simulink model "case7"  (R2024b)
settings: Solver=FixedStepAuto  StartTime=0  StopTime=1  FixedStep=1e-7  RelTol=1e-3
values from neighbouring files (symbols this model uses):
  SG_D_1_D = 0.01056    [IEEE9_case_parameters.m]    (also in case1_parameters.m; case2_parameters.m; case3_parameters.m; case4_parameters.m)
  SG_D_1_EnableSaturation = 0    [IEEE9_case_parameters.m]    (also in case1_parameters.m; case2_parameters.m; case3_parameters.m; case4_parameters.m)
  SG_D_1_f0 = 60    [IEEE9_case_parameters.m]    (also in case1_parameters.m; case2_parameters.m; case3_parameters.m; case4_parameters.m)
  SG_D_1_H = 7.5    [IEEE9_case_parameters.m]    (also in case1_parameters.m; case2_parameters.m; case3_parameters.m; case4_parameters.m)
  SG_D_1_K_A = 20    [IEEE9_case_parameters.m]    (also in case1_parameters.m; case2_parameters.m; case3_parameters.m; case4_parameters.m)
  SG_D_1_K_E = 1.000000e+1    (= 10)    [IEEE9_case_parameters.m]    (also in case1_parameters.m; case2_parameters.m; case3_parameters.m; case4_parameters.m)
  SG_D_1_K_F = 2.363    [IEEE9_case_parameters.m]    (also in case1_parameters.m; case2_parameters.m; case3_parameters.m; case4_parameters.m)
  SG_D_1_K_s = 0.5    [IEEE9_case_parameters.m]    (also in case1_parameters.m = 5; case2_parameters.m = 5; case3_parameters.m = 5; case4_parameters.m = 5)
  SG_D_1_R_a = 0.001088    [IEEE9_case_parameters.m]    (also in case1_parameters.m; case2_parameters.m; case3_parameters.m; case4_parameters.m)
  SG_D_1_S_A = 1    [IEEE9_case_parameters.m]    (also in case1_parameters.m; case2_parameters.m; case3_parameters.m; case4_parameters.m)
  SG_D_1_S_B = 0.103    [IEEE9_case_parameters.m]    (also in case1_parameters.m; case2_parameters.m; case3_parameters.m; case4_parameters.m)
  SG_D_1_S_N = 10.659857    [IEEE9_case_parameters.m]    (also in case1_parameters.m; case2_parameters.m; case3_parameters.m; case4_parameters.m)
  SG_D_1_SpeedPara = 200    [IEEE9_case_parameters.m]    (also in case1_parameters.m; case2_parameters.m; case3_parameters.m; case4_parameters.m)
  SG_D_1_T_0 = 0.720173    [IEEE9_case_parameters.m]    (also in case1_parameters.m = 0.755522; case2_parameters.m = 0.808931; case3_parameters.m = 0.869402; case4_parameters.m = 0.729316)
  SG_D_1_T_1 = 0.3    [IEEE9_case_parameters.m]    (also in case1_parameters.m; case2_parameters.m; case3_parameters.m; case4_parameters.m)
  SG_D_1_T_2 = 0.05    [IEEE9_case_parameters.m]    (also in case1_parameters.m; case2_parameters.m; case3_parameters.m; case4_parameters.m)
  SG_D_1_T_3 = 0.02    [IEEE9_case_parameters.m]    (also in case1_parameters.m; case2_parameters.m; case3_parameters.m; case4_parameters.m)
  SG_D_1_T_4 = 0.005    [IEEE9_case_parameters.m]    (also in case1_parameters.m; case2_parameters.m; case3_parameters.m; case4_parameters.m)
  SG_D_1_T_A = 0.02    [IEEE9_case_parameters.m]    (also in case1_parameters.m; case2_parameters.m; case3_parameters.m; case4_parameters.m)
  SG_D_1_T_dd = 8.000000e+0    (= 8)    [IEEE9_case_parameters.m]    (also in case1_parameters.m; case2_parameters.m; case3_parameters.m; case4_parameters.m)
  SG_D_1_T_ddd = 0.04    [IEEE9_case_parameters.m]    (also in case1_parameters.m; case2_parameters.m; case3_parameters.m; case4_parameters.m)
  SG_D_1_T_E = 0.314    [IEEE9_case_parameters.m]    (also in case1_parameters.m; case2_parameters.m; case3_parameters.m; case4_parameters.m)
  SG_D_1_T_F = 0.35    [IEEE9_case_parameters.m]    (also in case1_parameters.m; case2_parameters.m; case3_parameters.m; case4_parameters.m)
  SG_D_1_T_qd = 0.8    [IEEE9_case_parameters.m]    (also in case1_parameters.m; case2_parameters.m; case3_parameters.m; case4_parameters.m)
  SG_D_1_T_qdd = 0.02    [IEEE9_case_parameters.m]    (also in case1_parameters.m; case2_parameters.m; case3_parameters.m; case4_parameters.m)
  SG_D_1_T_speed = 0.1    [IEEE9_case_parameters.m]    (also in case1_parameters.m = 200; case2_parameters.m = 200; case3_parameters.m = 200; case4_parameters.m = 200)
  SG_D_1_T_w = 0.5    [IEEE9_case_parameters.m]    (also in case1_parameters.m; case2_parameters.m; case3_parameters.m; case4_parameters.m)
  SG_D_1_V_ref = 1.990276    [IEEE9_case_parameters.m]    (also in case1_parameters.m = 2.042296; case2_parameters.m = 2.051388; case3_parameters.m = 2.089584; case4_parameters.m = 2.01845)
  SG_D_1_w_ref = 376.991118    [IEEE9_case_parameters.m]    (also in case1_parameters.m; case2_parameters.m; case3_parameters.m; case4_parameters.m)
  SG_D_1_wb = 6.000000e+1    (= 60)    [IEEE9_case_parameters.m]    (also in case1_parameters.m; case2_parameters.m; case3_parameters.m; case4_parameters.m)
  SG_D_1_x_d = 1.9    [IEEE9_case_parameters.m]    (also in case1_parameters.m; case2_parameters.m; case3_parameters.m; case4_parameters.m)
  SG_D_1_x_dd = 0.302    [IEEE9_case_parameters.m]    (also in case1_parameters.m; case2_parameters.m; case3_parameters.m; case4_parameters.m)
  SG_D_1_x_ddd = 0.204    [IEEE9_case_parameters.m]    (also in case1_parameters.m; case2_parameters.m; case3_parameters.m; case4_parameters.m)
  SG_D_1_x_l = 0.05    [IEEE9_case_parameters.m]    (also in case1_parameters.m; case2_parameters.m; case3_parameters.m; case4_parameters.m)
  SG_D_1_x_q = 1.3    [IEEE9_case_parameters.m]    (also in case1_parameters.m; case2_parameters.m; case3_parameters.m; case4_parameters.m)
  SG_D_1_x_qd = 0.5    [IEEE9_case_parameters.m]    (also in case1_parameters.m; case2_parameters.m; case3_parameters.m; case4_parameters.m)
  SG_D_1_x_qdd = 0.3    [IEEE9_case_parameters.m]    (also in case1_parameters.m; case2_parameters.m; case3_parameters.m; case4_parameters.m)
  SG_D_2_D = 0.02    [IEEE9_case_parameters.m]    (also in case1_parameters.m; case2_parameters.m; case3_parameters.m; case4_parameters.m)
  SG_D_2_EnableSaturation = 0    [IEEE9_case_parameters.m]    (also in case1_parameters.m; case2_parameters.m; case3_parameters.m; case4_parameters.m)
  SG_D_2_f0 = 60    [IEEE9_case_parameters.m]    (also in case1_parameters.m; case2_parameters.m; case3_parameters.m; case4_parameters.m)
  SG_D_2_H = 8.000000e+0    (= 8)    [IEEE9_case_parameters.m]    (also in case1_parameters.m; case2_parameters.m; case3_parameters.m; case4_parameters.m)
  SG_D_2_K_A = 20    [IEEE9_case_parameters.m]    (also in case1_parameters.m; case2_parameters.m; case3_parameters.m; case4_parameters.m)
  SG_D_2_K_E = 1.000000e+1    (= 10)    [IEEE9_case_parameters.m]    (also in case1_parameters.m; case2_parameters.m; case3_parameters.m; case4_parameters.m)
  SG_D_2_K_F = 2.363    [IEEE9_case_parameters.m]    (also in case1_parameters.m; case2_parameters.m; case3_parameters.m; case4_parameters.m)
  SG_D_2_K_s = 0.5    [IEEE9_case_parameters.m]    (also in case1_parameters.m = 4; case2_parameters.m = 4; case3_parameters.m = 4; case4_parameters.m = 4)
  SG_D_2_R_a = 0.001088    [IEEE9_case_parameters.m]    (also in case1_parameters.m; case2_parameters.m; case3_parameters.m; case4_parameters.m)
  SG_D_2_S_A = 1    [IEEE9_case_parameters.m]    (also in case1_parameters.m; case2_parameters.m; case3_parameters.m; case4_parameters.m)
  SG_D_2_S_B = 0.103    [IEEE9_case_parameters.m]    (also in case1_parameters.m; case2_parameters.m; case3_parameters.m; case4_parameters.m)
  SG_D_2_S_N = 10.659857    [IEEE9_case_parameters.m]    (also in case1_parameters.m; case2_parameters.m; case3_parameters.m; case4_parameters.m)
  SG_D_2_SpeedPara = 200    [IEEE9_case_parameters.m]    (also in case1_parameters.m; case2_parameters.m; case3_parameters.m; case4_parameters.m)
  SG_D_2_T_0 = 1.632913    [IEEE9_case_parameters.m]    (also in case1_parameters.m = 1.632925; case2_parameters.m = 1.632915; case3_parameters.m = 1.632914; case4_parameters.m = 1.632927)
  SG_D_2_T_1 = 0.2    [IEEE9_case_parameters.m]    (also in case1_parameters.m; case2_parameters.m; case3_parameters.m; case4_parameters.m)
  SG_D_2_T_2 = 0.05    [IEEE9_case_parameters.m]    (also in case1_parameters.m; case2_parameters.m; case3_parameters.m; case4_parameters.m)
  SG_D_2_T_3 = 0.02    [IEEE9_case_parameters.m]    (also in case1_parameters.m; case2_parameters.m; case3_parameters.m; case4_parameters.m)
  SG_D_2_T_4 = 0.005    [IEEE9_case_parameters.m]    (also in case1_parameters.m; case2_parameters.m; case3_parameters.m; case4_parameters.m)
  SG_D_2_T_A = 0.02    [IEEE9_case_parameters.m]    (also in case1_parameters.m; case2_parameters.m; case3_parameters.m; case4_parameters.m)
  SG_D_2_T_dd = 7.9    [IEEE9_case_parameters.m]    (also in case1_parameters.m; case2_parameters.m; case3_parameters.m; case4_parameters.m)
  SG_D_2_T_ddd = 0.04    [IEEE9_case_parameters.m]    (also in case1_parameters.m; case2_parameters.m; case3_parameters.m; case4_parameters.m)
  SG_D_2_T_E = 0.314    [IEEE9_case_parameters.m]    (also in case1_parameters.m; case2_parameters.m; case3_parameters.m; case4_parameters.m)
  SG_D_2_T_F = 0.35    [IEEE9_case_parameters.m]    (also in case1_parameters.m; case2_parameters.m; case3_parameters.m; case4_parameters.m)
  SG_D_2_T_qd = 0.8    [IEEE9_case_parameters.m]    (also in case1_parameters.m; case2_parameters.m; case3_parameters.m; case4_parameters.m)
  SG_D_2_T_qdd = 0.015    [IEEE9_case_parameters.m]    (also in case1_parameters.m; case2_parameters.m; case3_parameters.m; case4_parameters.m)
  SG_D_2_T_speed = 0.1    [IEEE9_case_parameters.m]    (also in case1_parameters.m = 150; case2_parameters.m = 150; case3_parameters.m = 150; case4_parameters.m = 150)
  SG_D_2_T_w = 0.35    [IEEE9_case_parameters.m]    (also in case1_parameters.m; case2_parameters.m; case3_parameters.m; case4_parameters.m)
  SG_D_2_V_ref = 2.58547    [IEEE9_case_parameters.m]    (also in case1_parameters.m = 2.597896; case2_parameters.m = 2.587136; case3_parameters.m = 2.586042; case4_parameters.m = 2.599679)
  SG_D_2_w_ref = 376.991118    [IEEE9_case_parameters.m]    (also in case1_parameters.m; case2_parameters.m; case3_parameters.m; case4_parameters.m)
  SG_D_2_wb = 6.000000e+1    (= 60)    [IEEE9_case_parameters.m]    (also in case1_parameters.m; case2_parameters.m; case3_parameters.m; case4_parameters.m)
  SG_D_2_x_d = 1.8    [IEEE9_case_parameters.m]    (also in case1_parameters.m; case2_parameters.m; case3_parameters.m; case4_parameters.m)
  SG_D_2_x_dd = 0.302    [IEEE9_case_parameters.m]    (also in case1_parameters.m; case2_parameters.m; case3_parameters.m; case4_parameters.m)
  SG_D_2_x_ddd = 0.204    [IEEE9_case_parameters.m]    (also in case1_parameters.m; case2_parameters.m; case3_parameters.m; case4_parameters.m)
  SG_D_2_x_l = 0.05    [IEEE9_case_parameters.m]    (also in case1_parameters.m; case2_parameters.m; case3_parameters.m; case4_parameters.m)
  SG_D_2_x_q = 1.25    [IEEE9_case_parameters.m]    (also in case1_parameters.m; case2_parameters.m; case3_parameters.m; case4_parameters.m)
  SG_D_2_x_qd = 0.5    [IEEE9_case_parameters.m]    (also in case1_parameters.m; case2_parameters.m; case3_parameters.m; case4_parameters.m)
  SG_D_2_x_qdd = 0.3    [IEEE9_case_parameters.m]    (also in case1_parameters.m; case2_parameters.m; case3_parameters.m; case4_parameters.m)
  SG_D_3_D = 0.02    [IEEE9_case_parameters.m]    (also in case1_parameters.m; case2_parameters.m; case3_parameters.m; case4_parameters.m)
  SG_D_3_EnableSaturation = 0    [IEEE9_case_parameters.m]    (also in case1_parameters.m; case2_parameters.m; case3_parameters.m; case4_parameters.m)
  SG_D_3_f0 = 60    [IEEE9_case_parameters.m]    (also in case1_parameters.m; case2_parameters.m; case3_parameters.m; case4_parameters.m)
  SG_D_3_H = 7.7    [IEEE9_case_parameters.m]    (also in case1_parameters.m; case2_parameters.m; case3_parameters.m; case4_parameters.m)
  SG_D_3_K_A = 20    [IEEE9_case_parameters.m]    (also in case1_parameters.m; case2_parameters.m; case3_parameters.m; case4_parameters.m)
  SG_D_3_K_E = 1.000000e+1    (= 10)    [IEEE9_case_parameters.m]    (also in case1_parameters.m; case2_parameters.m; case3_parameters.m; case4_parameters.m)
  SG_D_3_K_F = 2.363    [IEEE9_case_parameters.m]    (also in case1_parameters.m; case2_parameters.m; case3_parameters.m; case4_parameters.m)
  SG_D_3_K_s = 0.2    [IEEE9_case_parameters.m]    (also in case1_parameters.m = 2; case2_parameters.m = 2; case3_parameters.m = 2; case4_parameters.m = 2)
  SG_D_3_R_a = 0.001088    [IEEE9_case_parameters.m]    (also in case1_parameters.m; case2_parameters.m; case3_parameters.m; case4_parameters.m)
  SG_D_3_S_A = 1    [IEEE9_case_parameters.m]    (also in case1_parameters.m; case2_parameters.m; case3_parameters.m; case4_parameters.m)
  SG_D_3_S_B = 0.103    [IEEE9_case_parameters.m]    (also in case1_parameters.m; case2_parameters.m; case3_parameters.m; case4_parameters.m)
  SG_D_3_S_N = 10.659857    [IEEE9_case_parameters.m]    (also in case1_parameters.m; case2_parameters.m; case3_parameters.m; case4_parameters.m)
  SG_D_3_SpeedPara = 200    [IEEE9_case_parameters.m]    (also in case1_parameters.m; case2_parameters.m; case3_parameters.m; case4_parameters.m)
  SG_D_3_T_0 = 0.850788    [IEEE9_case_parameters.m]    (also in case1_parameters.m = 0.850786; case2_parameters.m = 0.850787; case3_parameters.m; case4_parameters.m = 0.850786)
  SG_D_3_T_1 = 0.2    [IEEE9_case_parameters.m]    (also in case1_parameters.m; case2_parameters.m; case3_parameters.m; case4_parameters.m)
  SG_D_3_T_2 = 0.05    [IEEE9_case_parameters.m]    (also in case1_parameters.m; case2_parameters.m; case3_parameters.m; case4_parameters.m)
  SG_D_3_T_3 = 0.02    [IEEE9_case_parameters.m]    (also in case1_parameters.m; case2_parameters.m; case3_parameters.m; case4_parameters.m)
  SG_D_3_T_4 = 0.005    [IEEE9_case_parameters.m]    (also in case1_parameters.m; case2_parameters.m; case3_parameters.m; case4_parameters.m)
  SG_D_3_T_A = 0.02    [IEEE9_case_parameters.m]    (also in case1_parameters.m; case2_parameters.m; case3_parameters.m; case4_parameters.m)
  SG_D_3_T_dd = 8.1    [IEEE9_case_parameters.m]    (also in case1_parameters.m; case2_parameters.m; case3_parameters.m; case4_parameters.m)
  SG_D_3_T_ddd = 0.04    [IEEE9_case_parameters.m]    (also in case1_parameters.m; case2_parameters.m; case3_parameters.m; case4_parameters.m)
  SG_D_3_T_E = 0.314    [IEEE9_case_parameters.m]    (also in case1_parameters.m; case2_parameters.m; case3_parameters.m; case4_parameters.m)
  SG_D_3_T_F = 0.35    [IEEE9_case_parameters.m]    (also in case1_parameters.m; case2_parameters.m; case3_parameters.m; case4_parameters.m)
  SG_D_3_T_qd = 0.8    [IEEE9_case_parameters.m]    (also in case1_parameters.m; case2_parameters.m; case3_parameters.m; case4_parameters.m)
  SG_D_3_T_qdd = 0.015    [IEEE9_case_parameters.m]    (also in case1_parameters.m; case2_parameters.m; case3_parameters.m; case4_parameters.m)
  SG_D_3_T_speed = 0.1    [IEEE9_case_parameters.m]    (also in case1_parameters.m = 180; case2_parameters.m = 180; case3_parameters.m = 180; case4_parameters.m = 180)
  SG_D_3_T_w = 0.4    [IEEE9_case_parameters.m]    (also in case1_parameters.m; case2_parameters.m; case3_parameters.m; case4_parameters.m)
  SG_D_3_V_ref = 1.892727    [IEEE9_case_parameters.m]    (also in case1_parameters.m = 1.906439; case2_parameters.m = 1.895535; case3_parameters.m = 1.892105; case4_parameters.m = 1.906598)
  SG_D_3_w_ref = 376.991118    [IEEE9_case_parameters.m]    (also in case1_parameters.m; case2_parameters.m; case3_parameters.m; case4_parameters.m)
  SG_D_3_wb = 6.000000e+1    (= 60)    [IEEE9_case_parameters.m]    (also in case1_parameters.m; case2_parameters.m; case3_parameters.m; case4_parameters.m)
  SG_D_3_x_d = 1.85    [IEEE9_case_parameters.m]    (also in case1_parameters.m; case2_parameters.m; case3_parameters.m; case4_parameters.m)
  SG_D_3_x_dd = 0.302    [IEEE9_case_parameters.m]    (also in case1_parameters.m; case2_parameters.m; case3_parameters.m; case4_parameters.m)
  SG_D_3_x_ddd = 0.204    [IEEE9_case_parameters.m]    (also in case1_parameters.m; case2_parameters.m; case3_parameters.m; case4_parameters.m)
  SG_D_3_x_l = 0.05    [IEEE9_case_parameters.m]    (also in case1_parameters.m; case2_parameters.m; case3_parameters.m; case4_parameters.m)
  SG_D_3_x_q = 1.2    [IEEE9_case_parameters.m]    (also in case1_parameters.m; case2_parameters.m; case3_parameters.m; case4_parameters.m)
  SG_D_3_x_qd = 0.5    [IEEE9_case_parameters.m]    (also in case1_parameters.m; case2_parameters.m; case3_parameters.m; case4_parameters.m)
  SG_D_3_x_qdd = 0.3    [IEEE9_case_parameters.m]    (also in case1_parameters.m; case2_parameters.m; case3_parameters.m; case4_parameters.m)
(part 10 of 12)

== system case7/SG_D_3/d_R_f_SG_D_3_block ==
  note: d_R_f_SG_D_3 in case7
      | $-\frac{R_{f,\mathrm{SG},D,3}-\frac{E_{\mathrm{fd},\mathrm{SG},D,3}\,K_{F}}{T_{F}}}{T_{F}}$
      | Automatically generated on 2025-10-31 19:26:15 .
  State_E_fd_SG_D_3_188a8 : Inport
  State_R_f_SG_D_3_2f1ad : Inport  Port=2
  Constant_K_F_9434f : Constant  Value=K_F
  Constant_T_F_18230 : Constant  Value=T_F
  Constant_T_F_c7223 : Constant  Value=T_F
  Divide_08e52 : Product  Inputs=*/
  Divide_ece77 : Product  Inputs=*/
  Product_fb4d4 : Product
  Subtract_7a8c5 : Sum  Inputs=+-
  Blockout_d_R_f_SG_D_3_e162d : Outport
  wires:
  State_E_fd_SG_D_3_188a8/1 -> Product_fb4d4/1
  Constant_T_F_18230/1 -> Divide_08e52/2
  Constant_K_F_9434f/1 -> Product_fb4d4/2
  Product_fb4d4/1 -> Divide_08e52/1
  Divide_08e52/1 -> Subtract_7a8c5/1
  State_R_f_SG_D_3_2f1ad/1 -> Subtract_7a8c5/2
  Subtract_7a8c5/1 -> Divide_ece77/1
  Constant_T_F_c7223/1 -> Divide_ece77/2
  Divide_ece77/1 -> Blockout_d_R_f_SG_D_3_e162d/1

== system case7/SG_D_3/d_T_m_SG_D_3_block ==
  note: d_T_m_SG_D_3 in case7
      | $-\frac{T_{m,\mathrm{SG},D,3}-T_{0}+\frac{\mathrm{SpeedPara}\,\left(w_{\mathrm{SG},D,3}-w_{\mathrm{ref}}\right)}{2\,f_{0}\,\pi }}{T_{\mathrm{speed}}}$
      | Automatically generated on 2025-10-31 19:26:03 .
  State_w_SG_D_3_b61f5 : Inport
  State_T_m_SG_D_3_9a3dd : Inport  Port=2
  Add_b223b : Sum
  Add_f344e : Sum
  Constant_-1_ae0aa : Constant  Value=-1
  Constant_2.0_01156 : Constant  Value=2.0
  Constant_SpeedPara_6bcfb : Constant  Value=SpeedPara
  Constant_T_0_48b2f : Constant  Value=T_0
  Constant_T_speed_9a81d : Constant  Value=T_speed
  Constant_f0_c1c8d : Constant  Value=f0
  Constant_pi_99d26 : Constant  Value=pi
  Constant_w_ref_b4e4b : Constant  Value=w_ref
  Divide_4e7af : Product  Inputs=*/
  Divide_d9cbe : Product  Inputs=*/
  Product_15443 : Product
  Product_3cab2 : Product
  Product_667b3 : Product
  Product_fd20e : Product
  Subtract_9bc0b : Sum  Inputs=+-
  Blockout_d_T_m_SG_D_3_419d3 : Outport
  wires:
  Constant_SpeedPara_6bcfb/1 -> Product_3cab2/1
  Constant_-1_ae0aa/1 -> Product_15443/1
  Constant_w_ref_b4e4b/1 -> Add_f344e/2
  State_w_SG_D_3_b61f5/1 -> Product_15443/2
  Constant_2.0_01156/1 -> Product_fd20e/1
  Product_15443/1 -> Add_f344e/1
  Constant_pi_99d26/1 -> Product_fd20e/2
  Add_f344e/1 -> Product_3cab2/2
  Product_fd20e/1 -> Product_667b3/1
  Constant_f0_c1c8d/1 -> Product_667b3/2
  Product_3cab2/1 -> Divide_d9cbe/1
  Product_667b3/1 -> Divide_d9cbe/2
  Divide_d9cbe/1 -> Add_b223b/1
  Constant_T_0_48b2f/1 -> Add_b223b/2
  Add_b223b/1 -> Subtract_9bc0b/1
  State_T_m_SG_D_3_9a3dd/1 -> Subtract_9bc0b/2
  Subtract_9bc0b/1 -> Divide_4e7af/1
  Constant_T_speed_9a81d/1 -> Divide_4e7af/2
  Divide_4e7af/1 -> Blockout_d_T_m_SG_D_3_419d3/1

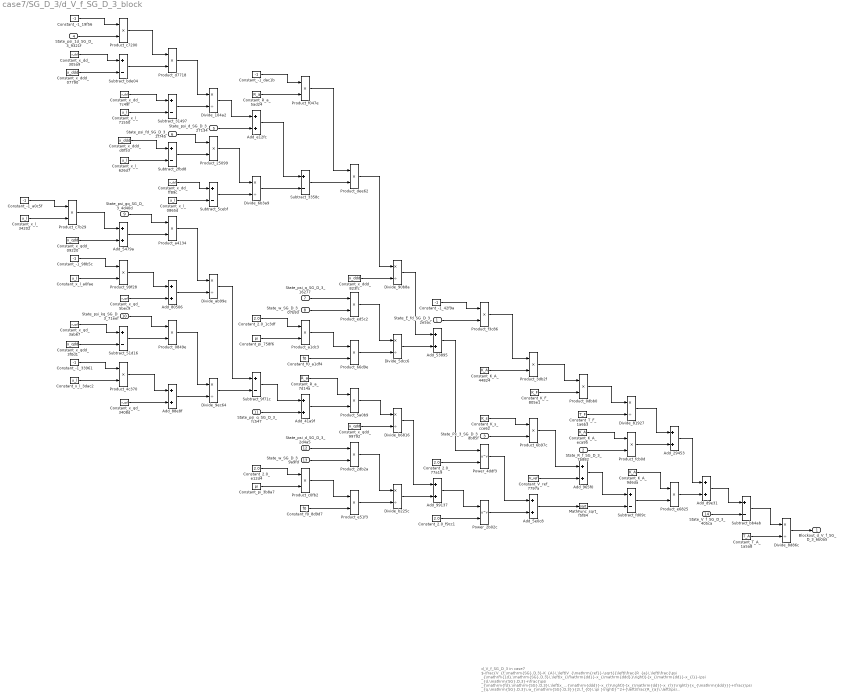
== system case7/SG_D_3/d_V_f_SG_D_3_block ==
  note: d_V_f_SG_D_3 in case7
      | $-\frac{V_{f,\mathrm{SG},D,3}-K_{A}\,\left(V_{\mathrm{ref}}-\sqrt{{\left(\frac{R_{a}\,\left(\frac{\psi _{\mathrm{1d},\mathrm{SG},D,3}\,\left(x_{\mathrm{dd}}-x_{\mathrm{ddd}}\right)}{x_{\mathrm{dd}}-x_{l}}-\psi _{d,\mathrm{SG},D,3}+\frac{\psi _{\mathrm{fd},\mathrm{SG},D,3}\,\left(x_{\mathrm{ddd}}-x_{l}\right)}{x_{\mathrm{dd}}-x_{l}}\right)}{x_{\mathrm{ddd}}}+\frac{\psi _{q,\mathrm{SG},D,3}\,w_{\mathrm{SG},D,3}}{2\,f_{0}\,\pi }\right)}^2+{\left(\frac{R_{a}\,\left(\psi _{q,\mathrm{SG},D,3}+\frac{\psi _{\mathrm{gq},\mathrm{SG},D,3}\,\left(x_{l}-x_{\mathrm{qdd}}\right)}{x_{l}-x_{\mathrm{qd}}}+\frac{\psi _{\mathrm{kq},\mathrm{SG},D,3}\,\left(x_{\mathrm{qd}}-x_{\mathrm{qdd}}\right)}{x_{l}-x_{\mathrm{qd}}}\right)}{x_{\mathrm{qdd}}}+\frac{\psi _{d,\mathrm{SG},D,3}\,w_{\mathrm{SG},D,3}}{2\,f_{0}\,\pi }\right)}^2}+K_{s}\,\mathrm{Px}_{3,\mathrm{SG},D,3}\right)-K_{A}\,R_{f,\mathrm{SG},D,3}+\frac{E_{\mathrm{fd},\mathrm{SG},D,3}\,K_{A}\,K_{F}}{T_{F}}}{T_{A}}$
      | Automatically generated on 2025-10-31 19:26:13 .
  State_E_fd_SG_D_3_2e5ac : Inport
  State_R_f_SG_D_3_7b882 : Inport  Port=2
  State_Px_3_SG_D_3_db85f : Inport  Port=3
  State_psi_1d_SG_D_3_9321f : Inport  Port=4
  State_psi_d_SG_D_3_27134 : Inport  Port=5
  State_psi_fd_SG_D_3_2f745 : Inport  Port=6
  State_psi_q_SG_D_3_16277 : Inport  Port=7
  State_w_SG_D_3_07b93 : Inport  Port=8
  State_psi_gq_SG_D_3_4d40d : Inport  Port=9
  State_psi_kq_SG_D_3_71eef : Inport  Port=10
  State_psi_q_SG_D_3_fc547 : Inport  Port=11
  State_psi_d_SG_D_3_2d4a5 : Inport  Port=12
  State_w_SG_D_3_9a9fd : Inport  Port=13
  State_V_f_SG_D_3_405ca : Inport  Port=14
  Add_{29453,53895,80506,99137} (4 alike) : Sum
  Add_41a9f : Sum
  Add_5479a : Sum
  Add_5e0c8 : Sum
  Add_88e8f : Sum
  Add_965f0 : Sum
  Add_d9e31 : Sum
  Add_e12fc : Sum
  Constant_-1_19f56 : Constant  Value=-1
  Constant_-1_33961 : Constant  Value=-1
  Constant_-1_42f9a : Constant  Value=-1
  Constant_-1_98b5c : Constant  Value=-1
  Constant_-1_a0c5f : Constant  Value=-1
  Constant_-1_dac1b : Constant  Value=-1
  Constant_2.0_1c3df : Constant  Value=2.0
  Constant_2.0_77a19 : Constant  Value=2.0
  Constant_2.0_e12d4 : Constant  Value=2.0
  Constant_2.0_f9cc1 : Constant  Value=2.0
  Constant_K_A_44824 : Constant  Value=K_A
  Constant_K_A_9d6da : Constant  Value=K_A
  Constant_K_A_eca95 : Constant  Value=K_A
  Constant_K_F_805e1 : Constant  Value=K_F
  Constant_K_s_cce62 : Constant  Value=K_s
  Constant_R_a_5ad24 : Constant  Value=R_a
  Constant_R_a_7d14a : Constant  Value=R_a
  Constant_T_A_1a5a8 : Constant  Value=T_A
  Constant_T_F_1a6b3 : Constant  Value=T_F
  Constant_V_ref_7797a : Constant  Value=V_ref
  Constant_f0_8d9d7 : Constant  Value=f0
  Constant_f0_a1df4 : Constant  Value=f0
  Constant_pi_3b8a7 : Constant  Value=pi
  Constant_pi_758f6 : Constant  Value=pi
  Constant_x_dd_305a9 : Constant  Value=x_dd
  Constant_x_dd_7c49f : Constant  Value=x_dd
  Constant_x_dd_ff89c : Constant  Value=x_dd
  Constant_x_ddd_07790 : Constant  Value=x_ddd
  Constant_x_ddd_823fc : Constant  Value=x_ddd
  Constant_x_ddd_d0f53 : Constant  Value=x_ddd
  Constant_x_l_0865d : Constant  Value=x_l
  Constant_x_l_34202 : Constant  Value=x_l
  Constant_x_l_3dac2 : Constant  Value=x_l
  Constant_x_l_626d7 : Constant  Value=x_l
  Constant_x_l_71550 : Constant  Value=x_l
  Constant_x_l_a0fae : Constant  Value=x_l
  Constant_x_qd_3408d : Constant  Value=x_qd
  Constant_x_qd_3ab67 : Constant  Value=x_qd
  Constant_x_qd_5bec9 : Constant  Value=x_qd
  Constant_x_qdd_09220 : Constant  Value=x_qdd
  Constant_x_qdd_3f0d1 : Constant  Value=x_qdd
  Constant_x_qdd_99792 : Constant  Value=x_qdd
  Divide_104a2 : Product  Inputs=*/
  Divide_5dcc6 : Product  Inputs=*/
  Divide_6b3a9 : Product  Inputs=*/
  Divide_81927 : Product  Inputs=*/
  Divide_8d86c : Product  Inputs=*/
  Divide_90b8a : Product  Inputs=*/
  Divide_9ec64 : Product  Inputs=*/
  Divide_ab99e : Product  Inputs=*/
  Divide_b225c : Product  Inputs=*/
  Divide_b6816 : Product  Inputs=*/
  MathFunc_sqrt_f5f84 : Sqrt
  Power_2b02c : Math  Operator=pow
  Power_4ddf3 : Math  Operator=pow
  Product_0849e : Product
  Product_0dbb0 : Product
  Product_25099 : Product
  Product_2db2a : Product
  Product_3db2f : Product
  Product_4c370 : Product
  Product_5a0b9 : Product
  Product_66d9e : Product
  Product_6b97c : Product
  Product_99f28 : Product
  Product_a1dc3 : Product
  Product_a4134 : Product
  Product_c0fb2 : Product
  Product_c7200 : Product
  Product_c7b29 : Product
  Product_d7718 : Product
  Product_dee62 : Product
  Product_e51f3 : Product
  Product_e6825 : Product
  Product_ed5c2 : Product
  Product_f047e : Product
  Product_f3c86 : Product
  Product_fcb0d : Product
  Subtract_2fbd8 : Sum  Inputs=+-
  Subtract_31497 : Sum  Inputs=+-
  Subtract_3358c : Sum  Inputs=+-
  Subtract_51d16 : Sum  Inputs=+-
  Subtract_5cebf : Sum  Inputs=+-
  Subtract_9f71c : Sum  Inputs=+-
  Subtract_bb4ab : Sum  Inputs=+-
  Subtract_bde04 : Sum  Inputs=+-
  Subtract_fd09c : Sum  Inputs=+-
  Blockout_d_V_f_SG_D_3_6b0a5 : Outport
  wires:
  Constant_K_A_eca95/1 -> Product_fcb0d/1
  Constant_-1_a0c5f/1 -> Product_c7b29/1
  Subtract_2fbd8/1 -> Product_25099/2
  Constant_x_l_34202/1 -> Product_c7b29/2
  Divide_b225c/1 -> Add_99137/2
  Constant_-1_19f56/1 -> Product_c7200/1
  State_psi_1d_SG_D_3_9321f/1 -> Product_c7200/2
  Constant_x_dd_305a9/1 -> Subtract_bde04/1
  Divide_6b3a9/1 -> Subtract_3358c/2
  Product_c7b29/1 -> Add_5479a/1
  Constant_x_qdd_09220/1 -> Add_5479a/2
  Constant_x_ddd_07790/1 -> Subtract_bde04/2
  Constant_2.0_f9cc1/1 -> Power_2b02c/2
  Constant_-1_98b5c/1 -> Product_99f28/1
  Divide_ab99e/1 -> Subtract_9f71c/1
  Subtract_31497/1 -> Divide_104a2/2
  Constant_x_l_a0fae/1 -> Product_99f28/2
  Constant_x_qd_3ab67/1 -> Subtract_51d16/1
  State_w_SG_D_3_07b93/1 -> Product_ed5c2/2
  Constant_x_qdd_3f0d1/1 -> Subtract_51d16/2
  Constant_2.0_1c3df/1 -> Product_a1dc3/1
  Constant_-1_33961/1 -> Product_4c370/1
  Constant_pi_758f6/1 -> Product_a1dc3/2
  Add_e12fc/1 -> Subtract_3358c/1
  Constant_x_l_3dac2/1 -> Product_4c370/2
  Product_c7200/1 -> Product_d7718/1
  Subtract_bde04/1 -> Product_d7718/2
  Constant_2.0_e12d4/1 -> Product_c0fb2/1
  Constant_x_dd_7c49f/1 -> Subtract_31497/1
  Constant_pi_3b8a7/1 -> Product_c0fb2/2
  Constant_x_l_71550/1 -> Subtract_31497/2
  Constant_x_ddd_d0f53/1 -> Subtract_2fbd8/1
  Constant_x_l_626d7/1 -> Subtract_2fbd8/2
  State_psi_gq_SG_D_3_4d40d/1 -> Product_a4134/1
  Constant_x_l_0865d/1 -> Subtract_5cebf/2
  Add_5479a/1 -> Product_a4134/2
  Product_99f28/1 -> Add_80506/1
  Product_a4134/1 -> Divide_ab99e/1
  Constant_x_qd_5bec9/1 -> Add_80506/2
  State_psi_kq_SG_D_3_71eef/1 -> Product_0849e/1
  State_psi_q_SG_D_3_16277/1 -> Product_ed5c2/1
  Add_53895/1 -> Power_4ddf3/1
  Subtract_51d16/1 -> Product_0849e/2
  Constant_f0_a1df4/1 -> Product_66d9e/2
  Product_a1dc3/1 -> Product_66d9e/1
  Constant_x_qd_3408d/1 -> Add_88e8f/2
  Product_4c370/1 -> Add_88e8f/1
  Product_d7718/1 -> Divide_104a2/1
  State_psi_fd_SG_D_3_2f745/1 -> Product_25099/1
  Constant_x_dd_ff89c/1 -> Subtract_5cebf/1
  Add_80506/1 -> Divide_ab99e/2
  Add_5e0c8/1 -> MathFunc_sqrt_f5f84/1
  Product_0849e/1 -> Divide_9ec64/1
  Add_88e8f/1 -> Divide_9ec64/2
  Product_f047e/1 -> Product_dee62/1
  Divide_104a2/1 -> Add_e12fc/1
  Add_965f0/1 -> Subtract_fd09c/1
  State_psi_d_SG_D_3_27134/1 -> Add_e12fc/2
  Product_25099/1 -> Divide_6b3a9/1
  Subtract_5cebf/1 -> Divide_6b3a9/2
  MathFunc_sqrt_f5f84/1 -> Subtract_fd09c/2
  Divide_9ec64/1 -> Subtract_9f71c/2
  Constant_-1_dac1b/1 -> Product_f047e/1
  Constant_R_a_5ad24/1 -> Product_f047e/2
  Subtract_9f71c/1 -> Add_41a9f/1
  State_psi_q_SG_D_3_fc547/1 -> Add_41a9f/2
  Subtract_3358c/1 -> Product_dee62/2
  Constant_R_a_7d14a/1 -> Product_5a0b9/1
  Add_41a9f/1 -> Product_5a0b9/2
  State_psi_d_SG_D_3_2d4a5/1 -> Product_2db2a/1
  State_w_SG_D_3_9a9fd/1 -> Product_2db2a/2
  Product_c0fb2/1 -> Product_e51f3/1
  Constant_f0_8d9d7/1 -> Product_e51f3/2
  Product_dee62/1 -> Divide_90b8a/1
  Constant_x_ddd_823fc/1 -> Divide_90b8a/2
  Product_ed5c2/1 -> Divide_5dcc6/1
  Product_66d9e/1 -> Divide_5dcc6/2
  Product_5a0b9/1 -> Divide_b6816/1
  Constant_x_qdd_99792/1 -> Divide_b6816/2
  Product_2db2a/1 -> Divide_b225c/1
  Product_e51f3/1 -> Divide_b225c/2
  Divide_90b8a/1 -> Add_53895/1
  Divide_5dcc6/1 -> Add_53895/2
  Divide_b6816/1 -> Add_99137/1
  Constant_-1_42f9a/1 -> Product_f3c86/1
  State_E_fd_SG_D_3_2e5ac/1 -> Product_f3c86/2
  Constant_2.0_77a19/1 -> Power_4ddf3/2
  Add_99137/1 -> Power_2b02c/1
  Product_f3c86/1 -> Product_3db2f/1
  Constant_K_A_44824/1 -> Product_3db2f/2
  Constant_K_s_cce62/1 -> Product_6b97c/1
  State_Px_3_SG_D_3_db85f/1 -> Product_6b97c/2
  Power_4ddf3/1 -> Add_5e0c8/1
  Power_2b02c/1 -> Add_5e0c8/2
  Product_3db2f/1 -> Product_0dbb0/1
  Constant_K_F_805e1/1 -> Product_0dbb0/2
  Product_6b97c/1 -> Add_965f0/1
  Constant_V_ref_7797a/1 -> Add_965f0/2
  Product_0dbb0/1 -> Divide_81927/1
  Constant_T_F_1a6b3/1 -> Divide_81927/2
  Add_d9e31/1 -> Subtract_bb4ab/1
  State_R_f_SG_D_3_7b882/1 -> Product_fcb0d/2
  Divide_81927/1 -> Add_29453/1
  Product_fcb0d/1 -> Add_29453/2
  Constant_K_A_9d6da/1 -> Product_e6825/1
  Subtract_fd09c/1 -> Product_e6825/2
  Add_29453/1 -> Add_d9e31/1
  Product_e6825/1 -> Add_d9e31/2
  State_V_f_SG_D_3_405ca/1 -> Subtract_bb4ab/2
  Subtract_bb4ab/1 -> Divide_8d86c/1
  Constant_T_A_1a5a8/1 -> Divide_8d86c/2
  Divide_8d86c/1 -> Blockout_d_V_f_SG_D_3_6b0a5/1

== system case7/SG_D_3/d_psi_1d_SG_D_3_block ==
  note: d_psi_1d_SG_D_3 in case7
      | $-\frac{\psi _{\mathrm{1d},\mathrm{SG},D,3}-\psi _{\mathrm{fd},\mathrm{SG},D,3}+\frac{\left(x_{\mathrm{dd}}-x_{l}\right)\,\left(\frac{\psi _{\mathrm{1d},\mathrm{SG},D,3}\,\left(x_{\mathrm{dd}}-x_{\mathrm{ddd}}\right)}{x_{\mathrm{dd}}-x_{l}}-\psi _{d,\mathrm{SG},D,3}+\frac{\psi _{\mathrm{fd},\mathrm{SG},D,3}\,\left(x_{\mathrm{ddd}}-x_{l}\right)}{x_{\mathrm{dd}}-x_{l}}\right)}{x_{\mathrm{ddd}}}}{T_{\mathrm{ddd}}}$
      | Automatically generated on 2025-10-31 19:25:51 .
  State_psi_1d_SG_D_3_0b4b8 : Inport
  State_psi_fd_SG_D_3_02f28 : Inport  Port=2
  State_psi_1d_SG_D_3_8936f : Inport  Port=3
  State_psi_d_SG_D_3_ea1f7 : Inport  Port=4
  State_psi_fd_SG_D_3_e1882 : Inport  Port=5
  Add_53690 : Sum
  Add_75a59 : Sum
  Add_8f410 : Sum
  Constant_-1_06d97 : Constant  Value=-1
  Constant_-1_0e0c1 : Constant  Value=-1
  Constant_T_ddd_7fe91 : Constant  Value=T_ddd
  Constant_x_dd_016c7 : Constant  Value=x_dd
  Constant_x_dd_0987d : Constant  Value=x_dd
  Constant_x_dd_21ef2 : Constant  Value=x_dd
  Constant_x_dd_adc50 : Constant  Value=x_dd
  Constant_x_ddd_1a67a : Constant  Value=x_ddd
  Constant_x_ddd_7c081 : Constant  Value=x_ddd
  Constant_x_ddd_b4a31 : Constant  Value=x_ddd
  Constant_x_l_81335 : Constant  Value=x_l
  Constant_x_l_97f1d : Constant  Value=x_l
  Constant_x_l_9c6ab : Constant  Value=x_l
  Constant_x_l_bed87 : Constant  Value=x_l
  Divide_843bb : Product  Inputs=*/
  Divide_c43ea : Product  Inputs=*/
  Divide_d9b03 : Product  Inputs=*/
  Divide_d9c08 : Product  Inputs=*/
  Product_1eb3f : Product
  Product_71d6f : Product
  Product_c74a5 : Product
  Product_d777a : Product
  Product_e7a17 : Product
  Subtract_51f62 : Sum  Inputs=+-
  Subtract_6497e : Sum  Inputs=+-
  Subtract_9d5e7 : Sum  Inputs=+-
  Subtract_9d617 : Sum  Inputs=+-
  Subtract_a4356 : Sum  Inputs=+-
  Subtract_ab385 : Sum  Inputs=+-
  Blockout_d_psi_1d_SG_D_3_24fb6 : Outport
  wires:
  Divide_d9c08/1 -> Add_53690/1
  Subtract_a4356/1 -> Product_e7a17/2
  Constant_-1_0e0c1/1 -> Product_d777a/1
  Constant_x_dd_adc50/1 -> Subtract_9d617/1
  State_psi_1d_SG_D_3_8936f/1 -> Product_d777a/2
  Product_d777a/1 -> Product_e7a17/1
  Constant_x_dd_21ef2/1 -> Subtract_a4356/1
  Constant_x_ddd_1a67a/1 -> Subtract_a4356/2
  Constant_x_l_9c6ab/1 -> Subtract_9d617/2
  Constant_x_ddd_7c081/1 -> Subtract_ab385/1
  Divide_d9b03/1 -> Blockout_d_psi_1d_SG_D_3_24fb6/1
  Constant_x_l_bed87/1 -> Subtract_ab385/2
  Product_e7a17/1 -> Divide_d9c08/1
  Subtract_9d617/1 -> Divide_d9c08/2
  State_psi_fd_SG_D_3_e1882/1 -> Product_71d6f/1
  Subtract_ab385/1 -> Product_71d6f/2
  Constant_x_dd_016c7/1 -> Subtract_51f62/1
  Constant_x_l_81335/1 -> Subtract_51f62/2
  State_psi_d_SG_D_3_ea1f7/1 -> Add_53690/2
  Product_71d6f/1 -> Divide_c43ea/1
  Subtract_51f62/1 -> Divide_c43ea/2
  Constant_x_dd_0987d/1 -> Subtract_9d5e7/1
  Constant_x_l_97f1d/1 -> Subtract_9d5e7/2
  Add_53690/1 -> Subtract_6497e/1
  Divide_c43ea/1 -> Subtract_6497e/2
  Constant_-1_06d97/1 -> Product_1eb3f/1
  State_psi_1d_SG_D_3_0b4b8/1 -> Product_1eb3f/2
  State_psi_fd_SG_D_3_02f28/1 -> Add_8f410/2
  Subtract_9d5e7/1 -> Product_c74a5/1
  Subtract_6497e/1 -> Product_c74a5/2
  Product_1eb3f/1 -> Add_8f410/1
  Product_c74a5/1 -> Divide_843bb/1
  Constant_x_ddd_b4a31/1 -> Divide_843bb/2
  Add_8f410/1 -> Add_75a59/1
  Divide_843bb/1 -> Add_75a59/2
  Add_75a59/1 -> Divide_d9b03/1
  Constant_T_ddd_7fe91/1 -> Divide_d9b03/2

== system case7/SG_D_3/d_psi_d_SG_D_3_block ==
  note: d_psi_d_SG_D_3 in case7
      | $2\,\pi \,f_{0}\,\left(v_{d,\mathrm{SG},D,3}\,\sin\left(\theta _{\mathrm{SG},D,3}\right)-v_{q,\mathrm{SG},D,3}\,\cos\left(\theta _{\mathrm{SG},D,3}\right)+\frac{R_{a}\,\left(\frac{\psi _{\mathrm{1d},\mathrm{SG},D,3}\,\left(x_{\mathrm{dd}}-x_{\mathrm{ddd}}\right)}{x_{\mathrm{dd}}-x_{l}}-\psi _{d,\mathrm{SG},D,3}+\frac{\psi _{\mathrm{fd},\mathrm{SG},D,3}\,\left(x_{\mathrm{ddd}}-x_{l}\right)}{x_{\mathrm{dd}}-x_{l}}\right)}{x_{\mathrm{ddd}}}+\frac{\psi _{q,\mathrm{SG},D,3}\,w_{\mathrm{SG},D,3}}{2\,f_{0}\,\pi }\right)$
      | Automatically generated on 2025-10-31 19:25:36 .
  State_psi_1d_SG_D_3_ab585 : Inport
  State_psi_d_SG_D_3_41343 : Inport  Port=2
  State_psi_fd_SG_D_3_7e2f5 : Inport  Port=3
  Input_v_d_SG_D_3_0a2ba : Inport  Port=4
  State_theta_SG_D_3_52860 : Inport  Port=5
  Input_v_q_SG_D_3_ba6ff : Inport  Port=6
  State_theta_SG_D_3_fae54 : Inport  Port=7
  State_psi_q_SG_D_3_1f0c4 : Inport  Port=8
  State_w_SG_D_3_0f458 : Inport  Port=9
  Add_26d2a : Sum
  Add_770bc : Sum
  Constant_-1_a0ac0 : Constant  Value=-1
  Constant_-2.0_c36db : Constant  Value=-2.0
  Constant_2.0_c736b : Constant  Value=2.0
  Constant_R_a_849c4 : Constant  Value=R_a
  Constant_f0_3d8b4 : Constant  Value=f0
  Constant_f0_94d50 : Constant  Value=f0
  Constant_pi_ef009 : Constant  Value=pi
  Constant_pi_fc779 : Constant  Value=pi
  Constant_x_dd_71fa9 : Constant  Value=x_dd
  Constant_x_dd_74ba0 : Constant  Value=x_dd
  Constant_x_dd_ba9eb : Constant  Value=x_dd
  Constant_x_ddd_2f5f8 : Constant  Value=x_ddd
  Constant_x_ddd_53176 : Constant  Value=x_ddd
  Constant_x_ddd_914c1 : Constant  Value=x_ddd
  Constant_x_l_43afa : Constant  Value=x_l
  Constant_x_l_5392c : Constant  Value=x_l
  Constant_x_l_d7c4e : Constant  Value=x_l
  Divide_0c0d1 : Product  Inputs=*/
  Divide_13e34 : Product  Inputs=*/
  Divide_90bb5 : Product  Inputs=*/
  Divide_d24ab : Product  Inputs=*/
  MathFunc_cos_a6b9c : Trigonometry  Operator=cos
  MathFunc_sin_06095 : Trigonometry
  Product_1ee4f : Product
  Product_3180b : Product
  Product_46370 : Product
  Product_535d4 : Product
  Product_63d43 : Product
  Product_6c6a9 : Product
  Product_83f5d : Product
  Product_8c848 : Product
  Product_8d27d : Product
  Product_a81cb : Product
  Product_b4903 : Product
  Product_c693f : Product
  Subtract_01828 : Sum  Inputs=+-
  Subtract_0f011 : Sum  Inputs=+-
  Subtract_2410f : Sum  Inputs=+-
  Subtract_28667 : Sum  Inputs=+-
  Subtract_40378 : Sum  Inputs=+-
  Subtract_72bdb : Sum  Inputs=+-
  Subtract_b37b2 : Sum  Inputs=+-
  Blockout_d_psi_d_SG_D_3_1dab3 : Outport
  wires:
  Constant_-1_a0ac0/1 -> Product_535d4/1
  Constant_2.0_c736b/1 -> Product_63d43/1
  Constant_x_dd_74ba0/1 -> Subtract_72bdb/1
  State_psi_1d_SG_D_3_ab585/1 -> Product_535d4/2
  Constant_x_dd_ba9eb/1 -> Subtract_0f011/1
  Constant_pi_ef009/1 -> Product_63d43/2
  Constant_x_ddd_53176/1 -> Subtract_72bdb/2
  Product_535d4/1 -> Product_b4903/1
  Product_63d43/1 -> Product_83f5d/1
  Subtract_72bdb/1 -> Product_b4903/2
  Constant_-2.0_c36db/1 -> Product_8c848/1
  Constant_x_l_5392c/1 -> Subtract_0f011/2
  Constant_x_ddd_2f5f8/1 -> Subtract_2410f/1
  Constant_pi_fc779/1 -> Product_8c848/2
  Constant_x_l_d7c4e/1 -> Subtract_2410f/2
  Product_3180b/1 -> Divide_0c0d1/1
  Product_b4903/1 -> Divide_13e34/1
  Subtract_0f011/1 -> Divide_13e34/2
  State_psi_fd_SG_D_3_7e2f5/1 -> Product_46370/1
  Subtract_2410f/1 -> Product_46370/2
  Constant_x_dd_71fa9/1 -> Subtract_40378/1
  Constant_x_l_43afa/1 -> Subtract_40378/2
  Divide_0c0d1/1 -> Subtract_28667/2
  Divide_13e34/1 -> Add_770bc/1
  Subtract_01828/1 -> Product_a81cb/2
  State_psi_d_SG_D_3_41343/1 -> Add_770bc/2
  Product_46370/1 -> Divide_90bb5/1
  Subtract_40378/1 -> Divide_90bb5/2
  Add_770bc/1 -> Subtract_01828/1
  Divide_90bb5/1 -> Subtract_01828/2
  Product_1ee4f/1 -> Add_26d2a/2
  Constant_R_a_849c4/1 -> Product_a81cb/1
  Product_8d27d/1 -> Product_c693f/1
  State_theta_SG_D_3_52860/1 -> MathFunc_sin_06095/1
  Product_a81cb/1 -> Divide_d24ab/1
  Constant_x_ddd_914c1/1 -> Divide_d24ab/2
  Input_v_d_SG_D_3_0a2ba/1 -> Product_6c6a9/1
  State_w_SG_D_3_0f458/1 -> Product_3180b/2
  MathFunc_sin_06095/1 -> Product_6c6a9/2
  State_theta_SG_D_3_fae54/1 -> MathFunc_cos_a6b9c/1
  MathFunc_cos_a6b9c/1 -> Product_1ee4f/2
  Divide_d24ab/1 -> Subtract_b37b2/1
  Product_6c6a9/1 -> Subtract_b37b2/2
  Input_v_q_SG_D_3_ba6ff/1 -> Product_1ee4f/1
  State_psi_q_SG_D_3_1f0c4/1 -> Product_3180b/1
  Constant_f0_3d8b4/1 -> Product_83f5d/2
  Subtract_b37b2/1 -> Add_26d2a/1
  Product_83f5d/1 -> Divide_0c0d1/2
  Product_8c848/1 -> Product_8d27d/1
  Constant_f0_94d50/1 -> Product_8d27d/2
  Add_26d2a/1 -> Subtract_28667/1
  Subtract_28667/1 -> Product_c693f/2
  Product_c693f/1 -> Blockout_d_psi_d_SG_D_3_1dab3/1

== system case7/SG_D_3/d_psi_fd_SG_D_3_block ==
  note: d_psi_fd_SG_D_3 in case7
      | $-\frac{\psi _{\mathrm{fd},\mathrm{SG},D,3}-E_{\mathrm{fd},\mathrm{SG},D,3}+\left(x_{d}-x_{\mathrm{dd}}\right)\,\left(\frac{\frac{\psi _{\mathrm{1d},\mathrm{SG},D,3}\,\left(x_{\mathrm{dd}}-x_{\mathrm{ddd}}\right)}{x_{\mathrm{dd}}-x_{l}}-\psi _{d,\mathrm{SG},D,3}+\frac{\psi _{\mathrm{fd},\mathrm{SG},D,3}\,\left(x_{\mathrm{ddd}}-x_{l}\right)}{x_{\mathrm{dd}}-x_{l}}}{x_{\mathrm{ddd}}}-\frac{\left(x_{\mathrm{dd}}-x_{\mathrm{ddd}}\right)\,\left(\psi _{\mathrm{1d},\mathrm{SG},D,3}-\psi _{\mathrm{fd},\mathrm{SG},D,3}+\frac{\left(x_{\mathrm{dd}}-x_{l}\right)\,\left(\frac{\psi _{\mathrm{1d},\mathrm{SG},D,3}\,\left(x_{\mathrm{dd}}-x_{\mathrm{ddd}}\right)}{x_{\mathrm{dd}}-x_{l}}-\psi _{d,\mathrm{SG},D,3}+\frac{\psi _{\mathrm{fd},\mathrm{SG},D,3}\,\left(x_{\mathrm{ddd}}-x_{l}\right)}{x_{\mathrm{dd}}-x_{l}}\right)}{x_{\mathrm{ddd}}}\right)}{{\left(x_{\mathrm{dd}}-x_{l}\right)}^2}\right)}{T_{\mathrm{dd}}}$
      | Automatically generated on 2025-10-31 19:25:47 .
  State_E_fd_SG_D_3_39d66 : Inport
  State_psi_fd_SG_D_3_d8879 : Inport  Port=2
  State_psi_1d_SG_D_3_05d9c : Inport  Port=3
  State_psi_fd_SG_D_3_36249 : Inport  Port=4
  State_psi_1d_SG_D_3_135f0 : Inport  Port=5
  State_psi_d_SG_D_3_e7d35 : Inport  Port=6
  State_psi_fd_SG_D_3_10381 : Inport  Port=7
  State_psi_1d_SG_D_3_2ff45 : Inport  Port=8
  State_psi_d_SG_D_3_5ac00 : Inport  Port=9
  State_psi_fd_SG_D_3_ba8dd : Inport  Port=10
  Add_35ec0 : Sum
  Add_d3d2a : Sum
  Constant_-1_04cd8 : Constant  Value=-1
  Constant_-1_5129c : Constant  Value=-1
  Constant_-1_f85fb : Constant  Value=-1
  Constant_2.0_d81cf : Constant  Value=2.0
  Constant_T_dd_ad31f : Constant  Value=T_dd
  Constant_x_d_9a0b5 : Constant  Value=x_d
  Constant_x_dd_206b0 : Constant  Value=x_dd
  Constant_x_dd_21bf2 : Constant  Value=x_dd
  Constant_x_dd_2e5c5 : Constant  Value=x_dd
  Constant_x_dd_86d43 : Constant  Value=x_dd
  Constant_x_dd_9b674 : Constant  Value=x_dd
  Constant_x_dd_a2618 : Constant  Value=x_dd
  Constant_x_dd_cc268 : Constant  Value=x_dd
  Constant_x_dd_d8ca3 : Constant  Value=x_dd
  Constant_x_dd_eb9ae : Constant  Value=x_dd
  Constant_x_dd_fcbea : Constant  Value=x_dd
  Constant_x_ddd_07501 : Constant  Value=x_ddd
  Constant_x_ddd_51c5a : Constant  Value=x_ddd
  Constant_x_ddd_6b385 : Constant  Value=x_ddd
  Constant_x_ddd_951f5 : Constant  Value=x_ddd
  Constant_x_ddd_b5ed7 : Constant  Value=x_ddd
  Constant_x_ddd_ddb46 : Constant  Value=x_ddd
  Constant_x_ddd_ee75d : Constant  Value=x_ddd
  Constant_x_l_15114 : Constant  Value=x_l
  Constant_x_l_45e7d : Constant  Value=x_l
  Constant_x_l_5314e : Constant  Value=x_l
  Constant_x_l_54785 : Constant  Value=x_l
  Constant_x_l_b62b7 : Constant  Value=x_l
  Constant_x_l_d7915 : Constant  Value=x_l
  Constant_x_l_f2beb : Constant  Value=x_l
  Constant_x_l_f539e : Constant  Value=x_l
  Divide_056ea : Product  Inputs=*/
  Divide_0c5fc : Product  Inputs=*/
  Divide_45999 : Product  Inputs=*/
  Divide_5afa3 : Product  Inputs=*/
  Divide_6ea7c : Product  Inputs=*/
  Divide_d2c8b : Product  Inputs=*/
  Divide_db002 : Product  Inputs=*/
  Divide_f1fcb : Product  Inputs=*/
  Power_ae863 : Math  Operator=pow
  Product_3caae : Product
  Product_4394e : Product
  Product_4403f : Product
  Product_4c687 : Product
  Product_5dfdd : Product
  Product_970f1 : Product
  Product_976a9 : Product
  Product_a5f0c : Product
  Product_e011b : Product
  Product_e6a7e : Product
  Subtract_1b4cd : Sum  Inputs=+-
  Subtract_214cc : Sum  Inputs=+-
  Subtract_2c21e : Sum  Inputs=+-
  Subtract_5a368 : Sum  Inputs=+-
  Subtract_5a536 : Sum  Inputs=+-
  Subtract_5ba41 : Sum  Inputs=+-
  Subtract_5ce01 : Sum  Inputs=+-
  Subtract_72162 : Sum  Inputs=+-
  Subtract_72ac6 : Sum  Inputs=+-
  Subtract_7a4e6 : Sum  Inputs=+-
  Subtract_825c6 : Sum  Inputs=+-
  Subtract_a0a76 : Sum  Inputs=+-
  Subtract_a2c3a : Sum  Inputs=+-
  Subtract_b959e : Sum  Inputs=+-
  Subtract_c2e19 : Sum  Inputs=+-
  Subtract_d1dc6 : Sum  Inputs=+-
  Subtract_e3631 : Sum  Inputs=+-
  Subtract_f0b4c : Sum  Inputs=+-
  Subtract_f2310 : Sum  Inputs=+-
  Blockout_d_psi_fd_SG_D_3_026a9 : Outport
  wires:
  Product_5dfdd/1 -> Divide_6ea7c/1
  Constant_-1_f85fb/1 -> Product_e011b/1
  Subtract_f2310/1 -> Product_976a9/2
  State_psi_1d_SG_D_3_135f0/1 -> Product_e011b/2
  Constant_x_l_54785/1 -> Subtract_1b4cd/2
  Constant_x_dd_21bf2/1 -> Subtract_f2310/1
  Constant_x_ddd_ee75d/1 -> Subtract_f2310/2
  Product_e011b/1 -> Product_976a9/1
  Constant_x_dd_cc268/1 -> Subtract_2c21e/1
  Constant_x_l_45e7d/1 -> Subtract_2c21e/2
  Constant_x_ddd_07501/1 -> Subtract_7a4e6/2
  Constant_x_ddd_51c5a/1 -> Subtract_214cc/1
  Constant_x_l_f2beb/1 -> Subtract_214cc/2
  Product_970f1/1 -> Product_3caae/1
  Product_976a9/1 -> Divide_f1fcb/1
  Subtract_2c21e/1 -> Divide_f1fcb/2
  State_psi_fd_SG_D_3_10381/1 -> Product_e6a7e/1
  Constant_x_ddd_951f5/1 -> Subtract_1b4cd/1
  Subtract_214cc/1 -> Product_e6a7e/2
  Constant_x_dd_9b674/1 -> Subtract_c2e19/1
  Constant_-1_5129c/1 -> Product_970f1/1
  Constant_x_l_5314e/1 -> Subtract_c2e19/2
  Product_3caae/1 -> Divide_5afa3/1
  Divide_f1fcb/1 -> Add_35ec0/1
  Product_4c687/1 -> Divide_0c5fc/1
  State_psi_d_SG_D_3_e7d35/1 -> Add_35ec0/2
  State_psi_fd_SG_D_3_ba8dd/1 -> Product_4c687/1
  Product_e6a7e/1 -> Divide_d2c8b/1
  Constant_x_dd_eb9ae/1 -> Subtract_b959e/1
  Subtract_c2e19/1 -> Divide_d2c8b/2
  Constant_x_l_d7915/1 -> Subtract_a0a76/2
  Constant_x_dd_2e5c5/1 -> Subtract_72162/1
  Subtract_5ce01/1 -> Product_4403f/2
  Constant_x_l_f539e/1 -> Subtract_72162/2
  Divide_5afa3/1 -> Add_d3d2a/1
  Constant_x_ddd_ddb46/1 -> Divide_6ea7c/2
  Add_35ec0/1 -> Subtract_5ba41/1
  Divide_d2c8b/1 -> Subtract_5ba41/2
  State_psi_1d_SG_D_3_2ff45/1 -> Product_970f1/2
  Constant_x_l_b62b7/1 -> Subtract_b959e/2
  Constant_x_dd_86d43/1 -> Subtract_7a4e6/1
  Subtract_72162/1 -> Product_5dfdd/1
  Add_d3d2a/1 -> Subtract_d1dc6/1
  Subtract_5ba41/1 -> Product_5dfdd/2
  Subtract_7a4e6/1 -> Product_3caae/2
  Constant_x_dd_206b0/1 -> Subtract_5a368/1
  Constant_x_l_15114/1 -> Subtract_5a368/2
  Subtract_1b4cd/1 -> Product_4c687/2
  Constant_x_dd_fcbea/1 -> Subtract_5ce01/1
  Constant_x_ddd_b5ed7/1 -> Subtract_5ce01/2
  Product_4403f/1 -> Product_4394e/1
  State_psi_1d_SG_D_3_05d9c/1 -> Subtract_a2c3a/1
  Subtract_5a368/1 -> Divide_5afa3/2
  State_psi_fd_SG_D_3_36249/1 -> Subtract_a2c3a/2
  Constant_-1_04cd8/1 -> Product_4403f/1
  Subtract_a2c3a/1 -> Subtract_5a536/1
  Divide_6ea7c/1 -> Subtract_5a536/2
  Constant_x_dd_a2618/1 -> Subtract_a0a76/1
  Divide_0c5fc/1 -> Subtract_d1dc6/2
  State_psi_d_SG_D_3_5ac00/1 -> Add_d3d2a/2
  Subtract_b959e/1 -> Divide_0c5fc/2
  Subtract_5a536/1 -> Product_4394e/2
  Subtract_a0a76/1 -> Power_ae863/1
  Constant_2.0_d81cf/1 -> Power_ae863/2
  Product_4394e/1 -> Divide_056ea/1
  Subtract_e3631/1 -> Product_a5f0c/2
  Power_ae863/1 -> Divide_056ea/2
  Subtract_d1dc6/1 -> Divide_db002/1
  Constant_x_ddd_6b385/1 -> Divide_db002/2
  Constant_x_d_9a0b5/1 -> Subtract_f0b4c/1
  Constant_x_dd_d8ca3/1 -> Subtract_f0b4c/2
  Divide_056ea/1 -> Subtract_e3631/1
  Divide_db002/1 -> Subtract_e3631/2
  State_E_fd_SG_D_3_39d66/1 -> Subtract_825c6/1
  State_psi_fd_SG_D_3_d8879/1 -> Subtract_825c6/2
  Subtract_f0b4c/1 -> Product_a5f0c/1
  Subtract_825c6/1 -> Subtract_72ac6/1
  Product_a5f0c/1 -> Subtract_72ac6/2
  Subtract_72ac6/1 -> Divide_45999/1
  Constant_T_dd_ad31f/1 -> Divide_45999/2
  Divide_45999/1 -> Blockout_d_psi_fd_SG_D_3_026a9/1
